simulink model "MR30Simulinknodos"  (R2013a)
settings: Solver=ode23tb  StartTime=0.0  StopTime=10.0  RelTol=1e-3
libraries: powerlib x200
(part 1 of 2)
settings Model: Creator=Erika  LastModifiedBy=Erika

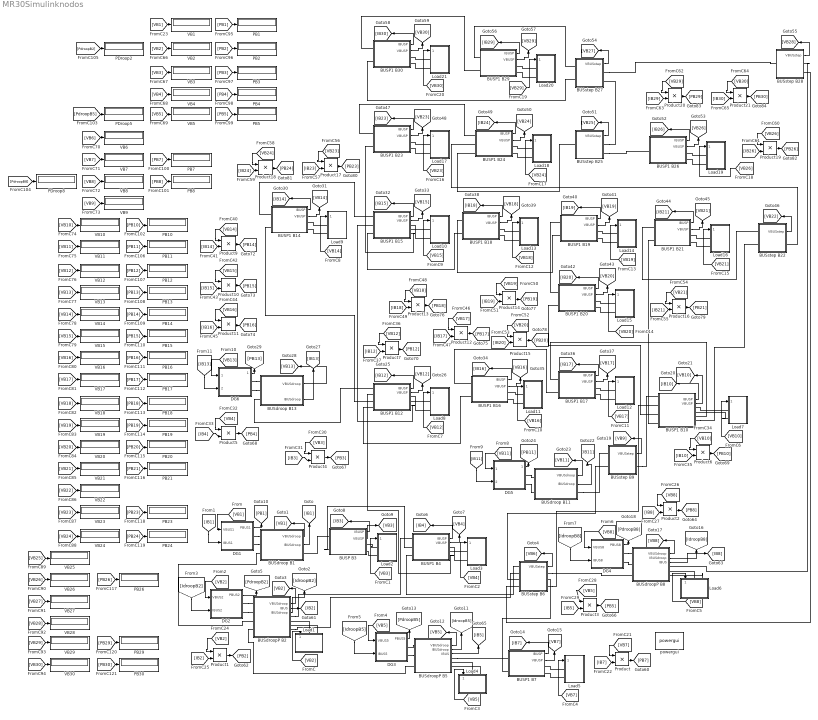
== system MR30Simulinknodos ==
  BUSP B3 : Subsystem
  BUSP1 B10 : Subsystem
  BUSP1 B12 : Subsystem
  BUSP1 B14 : Subsystem
  BUSP1 B15 : Subsystem
  BUSP1 B16 : Subsystem
  BUSP1 B17 : Subsystem
  BUSP1 B18 : Subsystem
  BUSP1 B19 : Subsystem
  BUSP1 B20 : Subsystem
  BUSP1 B21 : Subsystem
  BUSP1 B23 : Subsystem
  BUSP1 B24 : Subsystem
  BUSP1 B26 : Subsystem
  BUSP1 B29 : Subsystem
  BUSP1 B30 : Subsystem
  BUSP1 B4 : Subsystem
  BUSP1 B7 : Subsystem
  BUSdroop B1 : Subsystem
  BUSdroop B11 : Subsystem
  BUSdroop B13 : Subsystem
  BUSdroopP B2 : Subsystem
  BUSdroopP B5 : Subsystem
  BUSdroopP B8 : Subsystem
  BUSstep B22 : Subsystem
  BUSstep B25 : Subsystem
  BUSstep B27 : Subsystem
  BUSstep B28 : Subsystem
  BUSstep B6 : Subsystem
  BUSstep B9 : Subsystem
  DG1 : Subsystem
  DG2 : Subsystem
  DG3 : Subsystem
  DG4 : Subsystem
  DG5 : Subsystem
  DG6 : Subsystem
  Load1 : Subsystem
  Load10 : Subsystem
  Load11 : Subsystem
  Load12 : Subsystem
  Load13 : Subsystem
  Load14 : Subsystem
  Load15 : Subsystem
  Load16 : Subsystem
  Load17 : Subsystem
  Load18 : Subsystem
  Load19 : Subsystem
  Load2 : Subsystem
  Load20 : Subsystem
  Load21 : Subsystem
  Load3 : Subsystem
  Load4 : Subsystem
  Load5 : Subsystem
  Load6 : Subsystem
  Load7 : Subsystem
  Load8 : Subsystem
  Load9 : Subsystem
  PB{1..5,7..8,10..21,23..24,26,29..30} (24 alike) : Display
  PDroop2 : Display
  PDroop5 : Display
  PDroop8 : Display
  Product{,1..7,9..21} (21 alike) : Product
  VB{1..30} (30 alike) : Display
  powergui : powerlib/powergui  Priority=1  SimulationMode=Continuous  SolverType=Tustin  SampleTime=50e-6  frequency=60  SPID=off  DisableSnubberDevices=off  DisableRonSwitches=off  DisableVfSwitches=off  SwTol=0  Interpol=off  DisplayEquations=off  frequencyindice=0  Pbase=100e6  ErrMax=1e-4  Iterations=50  UnitsV=kV  UnitsW=MW  FunctionMessages=off  echomessages=off  HookPort=off  EnableUseOfTLC=off  x0status=blocks  RestoreLinks=warning  ResistiveCurrentMeasurement=off  Frange=[0:2:500]  Ylog=off  Xlog=on  ShowGrid=off  save=off  variable=ZData  ZoomFFT=off  StartTime=0.0  cycles=1  DisplayStyle=1  fundamental=60  FreqAxis=off  MaxFrequency=1000  frequencyindicesteady=1  RmsSteady=1  display=off  Ts=0  methode=off
  wires:
  BUSdroop B1/1(VBUSdroop) -> [VB1]
  BUSdroop B1/2(IBUSdroop) -> [IB1]
  [VB1] -> DG1/1(VBUS1)
  DG1/1(PBUS1) -> [PB1]
  BUSP B3/1(IBUSP) -> [IB3]
  BUSP B3/2(VBUSP) -> [VB3]
  [VB2] -> Load1/1(VBUSc)
  BUSdroopP B2/1(VBUSdroop) -> [VB2]
  BUSstep B6/1(VBUSstep) -> [VB6]
  [VB2] -> DG2/1(VBUS2)
  [IdroopB2] -> DG2/2(IBUS2)
  [VB3] -> Load2/1(VBUSc)
  BUSP1 B4/1(IBUSP) -> [IB4]
  BUSP1 B4/2(VBUSP) -> [VB4]
  [VB4] -> Load3/1(VBUSc)
  [VB5] -> Load4/1(VBUSc)
  BUSdroopP B5/1(VBUSdroop) -> [VB5]
  BUSdroopP B5/2(IBUSdroop) -> [IdroopB5]
  [VB5] -> DG3/1(VBUS5)
  [IdroopB5] -> DG3/2(IBUS5)
  DG3/1(PBUS5) -> [PdroopB5]
  BUSP1 B7/1(IBUSP) -> [IB7]
  BUSP1 B7/2(VBUSP) -> [VB7]
  [VB7] -> Load5/1(VBUSc)
  [VB8] -> Load6/1(VBUSc)
  BUSdroopP B8/1(VBUSdroop) -> [VB8]
  BUSdroopP B8/2(IBUSdroop) -> [IdroopB8]
  [VB8] -> DG4/1(VBUS8)
  [IdroopB8] -> DG4/2(IBUS8)
  DG4/1(PBUS8) -> [PdroopB8]
  BUSstep B9/1(VBUSstep) -> [VB9]
  BUSP1 B10/1(IBUSP) -> [IB10]
  BUSP1 B10/2(VBUSP) -> [VB10]
  [VB10] -> Load7/1(VBUSc)
  BUSdroop B11/1(VBUSdroop) -> [VB11]
  BUSdroop B11/2(IBUSdroop) -> [IB11]
  [VB11] -> DG5/1(VBUS11)
  [IB11] -> DG5/2(IBUS11)
  DG5/1(PBUS11) -> [PB11]
  BUSP1 B12/1(IBUSP) -> [IB12]
  BUSP1 B12/2(VBUSP) -> [VB12]
  [VB12] -> Load8/1(VBUSc)
  BUSdroop B13/1(VBUSdroop) -> [VB13]
  BUSdroop B13/2(IBUSdroop) -> [IB13]
  [VB13] -> DG6/1(VBUS13)
  [IB13] -> DG6/2(IBUS13)
  DG6/1(PBUS13) -> [PB13]
  BUSP1 B14/1(IBUSP) -> [IB14]
  BUSP1 B14/2(VBUSP) -> [VB14]
  [VB14] -> Load9/1(VBUSc)
  BUSP1 B15/1(IBUSP) -> [IB15]
  BUSP1 B15/2(VBUSP) -> [VB15]
  [VB15] -> Load10/1(VBUSc)
  BUSP1 B16/1(IBUSP) -> [IB16]
  BUSP1 B16/2(VBUSP) -> [VB16]
  [VB16] -> Load11/1(VBUSc)
  BUSP1 B17/1(IBUSP) -> [IB17]
  BUSP1 B17/2(VBUSP) -> [VB17]
  [VB17] -> Load12/1(VBUSc)
  BUSP1 B18/1(IBUSP) -> [IB18]
  BUSP1 B18/2(VBUSP) -> [VB18]
  [VB18] -> Load13/1(VBUSc)
  BUSP1 B19/1(IBUSP) -> [IB19]
  BUSP1 B19/2(VBUSP) -> [VB19]
  [VB19] -> Load14/1(VBUSc)
  BUSP1 B20/1(IBUSP) -> [IB20]
  BUSP1 B20/2(VBUSP) -> [VB20]
  [VB20] -> Load15/1(VBUSc)
  BUSP1 B21/1(IBUSP) -> [IB21]
  BUSP1 B21/2(VBUSP) -> [VB21]
  [VB21] -> Load16/1(VBUSc)
  BUSstep B22/1(VBUSstep) -> [VB22]
  BUSP1 B23/1(IBUSP) -> [IB23]
  BUSP1 B23/2(VBUSP) -> [VB23]
  [VB23] -> Load17/1(VBUSc)
  BUSP1 B24/1(IBUSP) -> [IB24]
  BUSP1 B24/2(VBUSP) -> [VB24]
  [VB24] -> Load18/1(VBUSc)
  BUSstep B25/1(VBUSstep) -> [VB25]
  BUSP1 B26/1(IBUSP) -> [IB26]
  BUSP1 B26/2(VBUSP) -> [VB26]
  [VB26] -> Load19/1(VBUSc)
  BUSstep B27/1(VBUSstep) -> [VB27]
  BUSstep B28/1(VBUSstep) -> [VB28]
  BUSP1 B29/1(IBUSP) -> [IB29]
  BUSP1 B29/2(VBUSP) -> [VB29]
  [VB29] -> Load20/1(VBUSc)
  BUSP1 B30/1(IBUSP) -> [IB30]
  BUSP1 B30/2(VBUSP) -> [VB30]
  [VB30] -> Load21/1(VBUSc)
  [IB1] -> DG1/2(IBUS1)
  Product/1 -> [PB7]
  [IB7] -> Product/2
  [VB7] -> Product/1
  DG2/1(PBUS2) -> [PdroopB2]
  Product1/1 -> [PB2]
  [IB2] -> Product1/2
  [VB2] -> Product1/1
  BUSdroopP B2/3(IBUSdroop) -> [IdroopB2]
  BUSdroopP B2/2(IBUS) -> [IB2]
  BUSdroopP B8/3(IBUS) -> [IB8]
  Product2/1 -> [PB8]
  [IB8] -> Product2/2
  [VB8] -> Product2/1
  BUSdroopP B5/3(IBUS) -> [IB5]
  Product3/1 -> [PB5]
  [IB5] -> Product3/2
  [VB5] -> Product3/1
  Product4/1 -> [PB3]
  [IB3] -> Product4/2
  [VB3] -> Product4/1
  Product5/1 -> [PB4]
  [IB4] -> Product5/2
  [VB4] -> Product5/1
  Product6/1 -> [PB10]
  [IB10] -> Product6/2
  [VB10] -> Product6/1
  Product7/1 -> [PB12]
  [IB12] -> Product7/2
  [VB12] -> Product7/1
  Product9/1 -> [PB14]
  [IB14] -> Product9/2
  [VB14] -> Product9/1
  Product10/1 -> [PB15]
  [IB15] -> Product10/2
  [VB15] -> Product10/1
  Product11/1 -> [PB16]
  [IB16] -> Product11/2
  [VB16] -> Product11/1
  Product12/1 -> [PB17]
  [IB17] -> Product12/2
  [VB17] -> Product12/1
  Product13/1 -> [PB18]
  [IB18] -> Product13/2
  [VB18] -> Product13/1
  Product14/1 -> [PB19]
  [IB19] -> Product14/2
  [VB19] -> Product14/1
  Product15/1 -> [PB20]
  [IB20] -> Product15/2
  [VB20] -> Product15/1
  Product16/1 -> [PB21]
  [IB21] -> Product16/2
  [VB21] -> Product16/1
  Product17/1 -> [PB23]
  [IB23] -> Product17/2
  [VB23] -> Product17/1
  Product18/1 -> [PB24]
  [IB24] -> Product18/2
  [VB24] -> Product18/1
  Product19/1 -> [PB26]
  [IB26] -> Product19/2
  [VB26] -> Product19/1
  Product20/1 -> [PB29]
  [IB29] -> Product20/2
  [VB29] -> Product20/1
  Product21/1 -> [PB30]
  [IB30] -> Product21/2
  [VB30] -> Product21/1
  [VB1] -> VB1/1
  [VB2] -> VB2/1
  [VB3] -> VB3/1
  [VB5] -> VB5/1
  [VB6] -> VB6/1
  [VB7] -> VB7/1
  [VB8] -> VB8/1
  [VB9] -> VB9/1
  [VB10] -> VB10/1
  [VB11] -> VB11/1
  [VB12] -> VB12/1
  [VB13] -> VB13/1
  [VB14] -> VB14/1
  [VB15] -> VB15/1
  [VB16] -> VB16/1
  [VB17] -> VB17/1
  [VB18] -> VB18/1
  [VB19] -> VB19/1
  [VB20] -> VB20/1
  [VB21] -> VB21/1
  [VB22] -> VB22/1
  [VB23] -> VB23/1
  [VB24] -> VB24/1
  [VB25] -> VB25/1
  [VB26] -> VB26/1
  [VB27] -> VB27/1
  [VB28] -> VB28/1
  [VB29] -> VB29/1
  [VB30] -> VB30/1
  [PB1] -> PB1/1
  [PB2] -> PB2/1
  [PB3] -> PB3/1
  [PB4] -> PB4/1
  [PB5] -> PB5/1
  [PB8] -> PB8/1
  [PB10] -> PB10/1
  [PdroopB5] -> PDroop5/1
  [PdroopB8] -> PDroop8/1
  [PdroopB2] -> PDroop2/1
  [PB12] -> PB12/1
  [PB13] -> PB13/1
  [PB14] -> PB14/1
  [PB15] -> PB15/1
  [PB16] -> PB16/1
  [PB17] -> PB17/1
  [PB18] -> PB18/1
  [PB19] -> PB19/1
  [PB20] -> PB20/1
  [PB21] -> PB21/1
  [PB23] -> PB23/1
  [PB24] -> PB24/1
  [PB26] -> PB26/1
  [PB29] -> PB29/1
  [PB30] -> PB30/1
  [PB11] -> PB11/1
  [PB7] -> PB7/1
  [VB4] -> VB4/1
  connections:
  DG1/RConn1 -- BUSdroop B1/LConn1
  DG1/RConn2 -- BUSdroop B1/LConn2
  DG2/RConn1 -- BUSdroopP B2/LConn1
  DG2/RConn2 -- BUSdroopP B2/LConn2
  Load1/LConn1 -- BUSdroopP B2/RConn2
  Load1/LConn2 -- BUSdroopP B2/RConn3
  Load2/LConn1 -- BUSP B3/RConn1
  Load2/LConn2 -- BUSP B3/RConn2
  Load3/LConn2 -- BUSP1 B4/RConn2
  Load3/LConn1 -- BUSP1 B4/RConn1
  DG3/RConn1 -- BUSdroopP B5/LConn1
  DG3/RConn2 -- BUSdroopP B5/LConn2
  Load4/LConn1 -- BUSdroopP B5/RConn2
  Load4/LConn2 -- BUSdroopP B5/RConn3
  Load5/LConn1 -- BUSP1 B7/RConn1
  Load5/LConn2 -- BUSP1 B7/RConn2
  Load6/LConn2 -- BUSdroopP B8/RConn3
  DG4/RConn1 -- BUSdroopP B8/LConn1
  DG4/RConn2 -- BUSdroopP B8/LConn2
  Load6/LConn1 -- BUSdroopP B8/RConn2
  Load7/LConn2 -- BUSP1 B10/RConn2
  Load7/LConn1 -- BUSP1 B10/RConn1
  DG5/RConn1 -- BUSdroop B11/LConn1
  DG5/RConn2 -- BUSdroop B11/LConn2
  Load8/LConn2 -- BUSP1 B12/RConn2
  Load8/LConn1 -- BUSP1 B12/RConn1
  DG6/RConn2 -- BUSdroop B13/LConn2
  DG6/RConn1 -- BUSdroop B13/LConn1
  Load9/LConn2 -- BUSP1 B14/RConn2
  Load9/LConn1 -- BUSP1 B14/RConn1
  Load10/LConn1 -- BUSP1 B15/RConn1
  Load10/LConn2 -- BUSP1 B15/RConn2
  Load11/LConn2 -- BUSP1 B16/RConn2
  Load11/LConn1 -- BUSP1 B16/RConn1
  Load12/LConn2 -- BUSP1 B17/RConn2
  Load12/LConn1 -- BUSP1 B17/RConn1
  Load13/LConn2 -- BUSP1 B18/RConn2
  Load13/LConn1 -- BUSP1 B18/RConn1
  Load14/LConn1 -- BUSP1 B19/RConn1
  Load14/LConn2 -- BUSP1 B19/RConn2
  Load15/LConn1 -- BUSP1 B20/RConn1
  Load15/LConn2 -- BUSP1 B20/RConn2
  Load16/LConn1 -- BUSP1 B21/RConn1
  Load16/LConn2 -- BUSP1 B21/RConn2
  Load17/LConn2 -- BUSP1 B23/RConn2
  Load17/LConn1 -- BUSP1 B23/RConn1
  Load18/LConn2 -- BUSP1 B24/RConn2
  Load18/LConn1 -- BUSP1 B24/RConn1
  Load19/LConn2 -- BUSP1 B26/RConn2
  Load19/LConn1 -- BUSP1 B26/RConn1
  Load20/LConn1 -- BUSP1 B29/RConn1
  Load20/LConn2 -- BUSP1 B29/RConn2
  Load21/LConn2 -- BUSP1 B30/RConn2
  Load21/LConn1 -- BUSP1 B30/RConn1
  BUSdroopP B2/LConn3 -- BUSdroop B1/LConn3
  BUSP B3/LConn1 -- BUSdroop B1/RConn1
  BUSdroopP B2/RConn1 -- BUSP1 B4/LConn1
  BUSP B3/LConn2 -- BUSP1 B4/LConn2
  BUSdroopP B2/LConn4 -- BUSdroopP B5/LConn3
  BUSdroopP B2/RConn4 -- BUSstep B6/LConn2
  BUSP1 B4/LConn3 -- BUSstep B6/LConn1
  BUSdroopP B5/RConn1 -- BUSP1 B7/LConn1
  BUSP1 B7/LConn2 -- BUSstep B6/RConn2
  BUSstep B6/RConn1 -- BUSdroopP B8/LConn3
  BUSstep B6/LConn3 -- BUSstep B9/LConn2
  BUSstep B6/RConn3 -- BUSP1 B10/LConn2
  BUSdroop B11/RConn1 -- BUSstep B9/LConn1
  BUSstep B9/RConn1 -- BUSP1 B10/LConn1
  BUSP1 B4/RConn3 -- BUSP1 B12/LConn2
  BUSdroop B13/LConn3 -- BUSP1 B12/LConn1
  BUSP1 B14/LConn2 -- BUSP1 B12/LConn3
  BUSP1 B12/RConn3 -- BUSP1 B15/LConn2
  BUSP1 B12/LConn4 -- BUSP1 B16/LConn2
  BUSP1 B14/LConn1 -- BUSP1 B15/LConn1
  BUSP1 B16/LConn1 -- BUSP1 B17/LConn2
  BUSP1 B15/LConn3 -- BUSP1 B18/LConn2
  BUSP1 B18/LConn1 -- BUSP1 B19/LConn2
  BUSP1 B20/LConn1 -- BUSP1 B19/LConn1
  BUSP1 B20/LConn2 -- BUSP1 B10/LConn3
  BUSP1 B17/LConn1 -- BUSP1 B10/RConn3
  BUSP1 B21/LConn2 -- BUSP1 B10/LConn4
  BUSP1 B10/RConn4 -- BUSstep B22/LConn2
  BUSP1 B21/LConn1 -- BUSstep B22/LConn1
  BUSP1 B15/RConn3 -- BUSP1 B23/LConn2
  BUSP1 B24/LConn2 -- BUSstep B22/RConn1
  BUSP1 B23/LConn1 -- BUSP1 B24/LConn1
  BUSP1 B24/LConn3 -- BUSstep B25/LConn1
  BUSstep B25/RConn2 -- BUSP1 B26/LConn1
  BUSstep B25/RConn1 -- BUSstep B27/RConn2
  BUSstep B27/RConn1 -- BUSstep B28/LConn1
  BUSstep B27/LConn1 -- BUSP1 B29/LConn1
  BUSP1 B30/LConn2 -- BUSstep B27/LConn2
  BUSP1 B30/LConn1 -- BUSP1 B29/LConn2
  BUSstep B28/RConn1 -- BUSdroopP B8/RConn1
  BUSstep B6/LConn4 -- BUSstep B28/RConn2

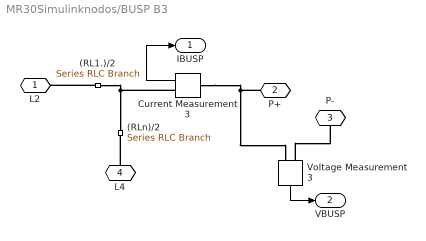
== system MR30Simulinknodos/BUSP B3 ==
  (RL1.)/2 : powerlib/Elements/Series RLC Branch  LConnTagsString=__new0  RConnTagsString=__new0  BranchType=R  Resistance=0.645456/2  Inductance=1e-3  SetiL0=off  InitialCurrent=0  Capacitance=1e-6  Setx0=off  InitialVoltage=0  Measurements=None
  (RLn)/2 : powerlib/Elements/Series RLC Branch  LConnTagsString=__new0  RConnTagsString=__new0  BranchType=R  Resistance=.188496/2  Inductance=1e-3  SetiL0=off  InitialCurrent=0  Capacitance=1e-6  Setx0=off  InitialVoltage=0  Measurements=None
  Current Measurement3 : powerlib/Measurements/Current Measurement  PhasorSimulation=off  OutputType=Complex  PSBequivalent=0
  Voltage Measurement3 : powerlib/Measurements/Voltage Measurement  PhasorSimulation=off  OutputType=Complex  PSBequivalent=0
  L2 : PMIOPort  Port=1  Side=Left
  P+ : PMIOPort  Port=2  Side=Right
  P- : PMIOPort  Port=3  Side=Right
  L4 : PMIOPort  Port=4  Side=Left
  IBUSP : Outport
  VBUSP : Outport  Port=2
  wires:
  Voltage Measurement3/1 -> VBUSP/1
  Current Measurement3/1 -> IBUSP/1
  connections:
  P+/RConn1 -- Voltage Measurement3/LConn1 -- Current Measurement3/LConn1
  (RL1.)/2/RConn1 -- Current Measurement3/RConn1 -- (RLn)/2/LConn1
  (RL1.)/2/LConn1 -- L2/RConn1
  L4/RConn1 -- (RLn)/2/RConn1
  Voltage Measurement3/LConn2 -- P-/RConn1

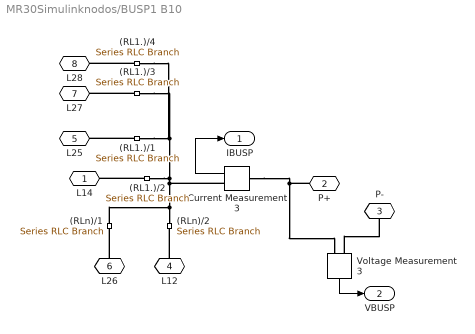
== system MR30Simulinknodos/BUSP1 B10 ==
  (RL1.)/1 : powerlib/Elements/Series RLC Branch  LConnTagsString=__new0  RConnTagsString=__new0  BranchType=R  Resistance=1.336608/2  Inductance=1e-3  SetiL0=off  InitialCurrent=0  Capacitance=1e-6  Setx0=off  InitialVoltage=0  Measurements=None
  (RL1.)/2 : powerlib/Elements/Series RLC Branch  LConnTagsString=__new0  RConnTagsString=__new0  BranchType=R  Resistance=1.5708/2  Inductance=1e-3  SetiL0=off  InitialCurrent=0  Capacitance=1e-6  Setx0=off  InitialVoltage=0  Measurements=None
  (RL1.)/3 : powerlib/Elements/Series RLC Branch  LConnTagsString=__new0  RConnTagsString=__new0  BranchType=R  Resistance=0.496944/2  Inductance=1e-3  SetiL0=off  InitialCurrent=0  Capacitance=1e-6  Setx0=off  InitialVoltage=0  Measurements=None
  (RL1.)/4 : powerlib/Elements/Series RLC Branch  LConnTagsString=__new0  RConnTagsString=__new0  BranchType=R  Resistance=1.038156/2  Inductance=1e-3  SetiL0=off  InitialCurrent=0  Capacitance=1e-6  Setx0=off  InitialVoltage=0  Measurements=None
  (RLn)/1 : powerlib/Elements/Series RLC Branch  LConnTagsString=__new0  RConnTagsString=__new0  BranchType=R  Resistance=0.462672/2  Inductance=1e-3  SetiL0=off  InitialCurrent=0  Capacitance=1e-6  Setx0=off  InitialVoltage=0  Measurements=None
  (RLn)/2 : powerlib/Elements/Series RLC Branch  LConnTagsString=__new0  RConnTagsString=__new0  BranchType=R  Resistance=7.93968/2  Inductance=1e-3  SetiL0=off  InitialCurrent=0  Capacitance=1e-6  Setx0=off  InitialVoltage=0  Measurements=None
  Current Measurement3 : powerlib/Measurements/Current Measurement  PhasorSimulation=off  OutputType=Complex  PSBequivalent=0
  Voltage Measurement3 : powerlib/Measurements/Voltage Measurement  PhasorSimulation=off  OutputType=Complex  PSBequivalent=0
  L14 : PMIOPort  Port=1  Side=Left
  P+ : PMIOPort  Port=2  Side=Right
  P- : PMIOPort  Port=3  Side=Right
  L12 : PMIOPort  Port=4  Side=Left
  L25 : PMIOPort  Port=5  Side=Left
  L26 : PMIOPort  Port=6  Side=Right
  L27 : PMIOPort  Port=7  Side=Left
  L28 : PMIOPort  Port=8  Side=Right
  IBUSP : Outport
  VBUSP : Outport  Port=2
  wires:
  Current Measurement3/1 -> IBUSP/1
  Voltage Measurement3/1 -> VBUSP/1
  connections:
  Voltage Measurement3/LConn2 -- P-/RConn1
  L12/RConn1 -- (RLn)/2/RConn1
  (RL1.)/2/LConn1 -- L14/RConn1
  (RL1.)/4/RConn1 -- (RL1.)/3/RConn1 -- (RL1.)/1/RConn1 -- (RL1.)/2/RConn1 -- Current Measurement3/RConn1 -- (RLn)/1/LConn1 -- (RLn)/2/LConn1
  Current Measurement3/LConn1 -- Voltage Measurement3/LConn1 -- P+/RConn1
  (RL1.)/1/LConn1 -- L25/RConn1
  L26/RConn1 -- (RLn)/1/RConn1
  (RL1.)/3/LConn1 -- L27/RConn1
  (RL1.)/4/LConn1 -- L28/RConn1

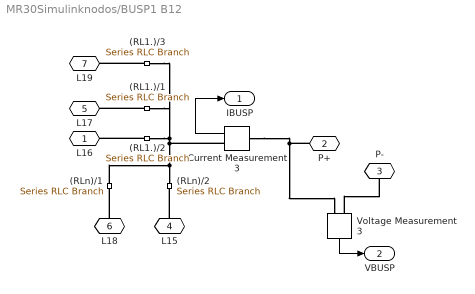
== system MR30Simulinknodos/BUSP1 B12 ==
  (RL1.)/1 : powerlib/Elements/Series RLC Branch  LConnTagsString=__new0  RConnTagsString=__new0  BranchType=R  Resistance=1.757868/2  Inductance=1e-3  SetiL0=off  InitialCurrent=0  Capacitance=1e-6  Setx0=off  InitialVoltage=0  Measurements=None
  (RL1.)/2 : powerlib/Elements/Series RLC Branch  LConnTagsString=__new0  RConnTagsString=__new0  BranchType=R  Resistance=1.9992/2  Inductance=1e-3  SetiL0=off  InitialCurrent=0  Capacitance=1e-6  Setx0=off  InitialVoltage=0  Measurements=None
  (RL1.)/3 : powerlib/Elements/Series RLC Branch  LConnTagsString=__new0  RConnTagsString=__new0  BranchType=R  Resistance=1.34946/2  Inductance=1e-3  SetiL0=off  InitialCurrent=0  Capacitance=1e-6  Setx0=off  InitialVoltage=0  Measurements=None
  (RLn)/1 : powerlib/Elements/Series RLC Branch  LConnTagsString=__new0  RConnTagsString=__new0  BranchType=R  Resistance=0.945336/2  Inductance=1e-3  SetiL0=off  InitialCurrent=0  Capacitance=1e-6  Setx0=off  InitialVoltage=0  Measurements=None
  (RLn)/2 : powerlib/Elements/Series RLC Branch  LConnTagsString=__new0  RConnTagsString=__new0  BranchType=R  Resistance=3.65568/2  Inductance=1e-3  SetiL0=off  InitialCurrent=0  Capacitance=1e-6  Setx0=off  InitialVoltage=0  Measurements=None
  Current Measurement3 : powerlib/Measurements/Current Measurement  PhasorSimulation=off  OutputType=Complex  PSBequivalent=0
  Voltage Measurement3 : powerlib/Measurements/Voltage Measurement  PhasorSimulation=off  OutputType=Complex  PSBequivalent=0
  L16 : PMIOPort  Port=1  Side=Left
  P+ : PMIOPort  Port=2  Side=Right
  P- : PMIOPort  Port=3  Side=Right
  L15 : PMIOPort  Port=4  Side=Left
  L17 : PMIOPort  Port=5  Side=Left
  L18 : PMIOPort  Port=6  Side=Right
  L19 : PMIOPort  Port=7  Side=Left
  IBUSP : Outport
  VBUSP : Outport  Port=2
  wires:
  Voltage Measurement3/1 -> VBUSP/1
  Current Measurement3/1 -> IBUSP/1
  connections:
  P+/RConn1 -- Voltage Measurement3/LConn1 -- Current Measurement3/LConn1
  (RL1.)/2/RConn1 -- (RL1.)/3/RConn1 -- (RL1.)/1/RConn1 -- Current Measurement3/RConn1 -- (RLn)/1/LConn1 -- (RLn)/2/LConn1
  (RL1.)/2/LConn1 -- L16/RConn1
  L15/RConn1 -- (RLn)/2/RConn1
  Voltage Measurement3/LConn2 -- P-/RConn1
  (RL1.)/1/LConn1 -- L17/RConn1
  L18/RConn1 -- (RLn)/1/RConn1
  (RL1.)/3/LConn1 -- L19/RConn1

== system MR30Simulinknodos/BUSP1 B14 ==
  (RL1.)/2 : powerlib/Elements/Series RLC Branch  LConnTagsString=__new0  RConnTagsString=__new0  BranchType=R  Resistance=3.15588/2  Inductance=1e-3  SetiL0=off  InitialCurrent=0  Capacitance=1e-6  Setx0=off  InitialVoltage=0  Measurements=None
  (RLn)/2 : powerlib/Elements/Series RLC Branch  LConnTagsString=__new0  RConnTagsString=__new0  BranchType=R  Resistance=1.757868/2  Inductance=1e-3  SetiL0=off  InitialCurrent=0  Capacitance=1e-6  Setx0=off  InitialVoltage=0  Measurements=None
  Current Measurement3 : powerlib/Measurements/Current Measurement  PhasorSimulation=off  OutputType=Complex  PSBequivalent=0
  Voltage Measurement3 : powerlib/Measurements/Voltage Measurement  PhasorSimulation=off  OutputType=Complex  PSBequivalent=0
  L20 : PMIOPort  Port=1  Side=Left
  P+ : PMIOPort  Port=2  Side=Right
  P- : PMIOPort  Port=3  Side=Right
  L17 : PMIOPort  Port=4  Side=Left
  IBUSP : Outport
  VBUSP : Outport  Port=2
  wires:
  Current Measurement3/1 -> IBUSP/1
  Voltage Measurement3/1 -> VBUSP/1
  connections:
  Voltage Measurement3/LConn2 -- P-/RConn1
  L17/RConn1 -- (RLn)/2/RConn1
  (RL1.)/2/LConn1 -- L20/RConn1
  (RLn)/2/LConn1 -- Current Measurement3/RConn1 -- (RL1.)/2/RConn1
  Current Measurement3/LConn1 -- Voltage Measurement3/LConn1 -- P+/RConn1

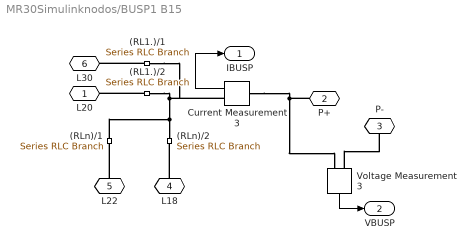
== system MR30Simulinknodos/BUSP1 B15 ==
  (RL1.)/1 : powerlib/Elements/Series RLC Branch  LConnTagsString=__new0  RConnTagsString=__new0  BranchType=R  Resistance=1.428/2  Inductance=1e-3  SetiL0=off  InitialCurrent=0  Capacitance=1e-6  Setx0=off  InitialVoltage=0  Measurements=None
  (RL1.)/2 : powerlib/Elements/Series RLC Branch  LConnTagsString=__new0  RConnTagsString=__new0  BranchType=R  Resistance=3.15588/2  Inductance=1e-3  SetiL0=off  InitialCurrent=0  Capacitance=1e-6  Setx0=off  InitialVoltage=0  Measurements=None
  (RLn)/1 : powerlib/Elements/Series RLC Branch  LConnTagsString=__new0  RConnTagsString=__new0  BranchType=R  Resistance=1.52796/2  Inductance=1e-3  SetiL0=off  InitialCurrent=0  Capacitance=1e-6  Setx0=off  InitialVoltage=0  Measurements=None
  (RLn)/2 : powerlib/Elements/Series RLC Branch  LConnTagsString=__new0  RConnTagsString=__new0  BranchType=R  Resistance=0.945336/2  Inductance=1e-3  SetiL0=off  InitialCurrent=0  Capacitance=1e-6  Setx0=off  InitialVoltage=0  Measurements=None
  Current Measurement3 : powerlib/Measurements/Current Measurement  PhasorSimulation=off  OutputType=Complex  PSBequivalent=0
  Voltage Measurement3 : powerlib/Measurements/Voltage Measurement  PhasorSimulation=off  OutputType=Complex  PSBequivalent=0
  L20 : PMIOPort  Port=1  Side=Left
  P+ : PMIOPort  Port=2  Side=Right
  P- : PMIOPort  Port=3  Side=Right
  L18 : PMIOPort  Port=4  Side=Left
  L22 : PMIOPort  Port=5  Side=Left
  L30 : PMIOPort  Port=6  Side=Right
  IBUSP : Outport
  VBUSP : Outport  Port=2
  wires:
  Voltage Measurement3/1 -> VBUSP/1
  Current Measurement3/1 -> IBUSP/1
  connections:
  P+/RConn1 -- Voltage Measurement3/LConn1 -- Current Measurement3/LConn1
  (RL1.)/2/RConn1 -- (RL1.)/1/RConn1 -- Current Measurement3/RConn1 -- (RLn)/1/LConn1 -- (RLn)/2/LConn1
  (RL1.)/2/LConn1 -- L20/RConn1
  L18/RConn1 -- (RLn)/2/RConn1
  Voltage Measurement3/LConn2 -- P-/RConn1
  L22/RConn1 -- (RLn)/1/RConn1
  (RL1.)/1/LConn1 -- L30/RConn1

== system MR30Simulinknodos/BUSP1 B16 ==
  (RL1.)/2 : powerlib/Elements/Series RLC Branch  LConnTagsString=__new0  RConnTagsString=__new0  BranchType=R  Resistance=1.176672/2  Inductance=1e-3  SetiL0=off  InitialCurrent=0  Capacitance=1e-6  Setx0=off  InitialVoltage=0  Measurements=None
  (RLn)/2 : powerlib/Elements/Series RLC Branch  LConnTagsString=__new0  RConnTagsString=__new0  BranchType=R  Resistance=1.34946/2  Inductance=1e-3  SetiL0=off  InitialCurrent=0  Capacitance=1e-6  Setx0=off  InitialVoltage=0  Measurements=None
  Current Measurement3 : powerlib/Measurements/Current Measurement  PhasorSimulation=off  OutputType=Complex  PSBequivalent=0
  Voltage Measurement3 : powerlib/Measurements/Voltage Measurement  PhasorSimulation=off  OutputType=Complex  PSBequivalent=0
  L21 : PMIOPort  Port=1  Side=Left
  P+ : PMIOPort  Port=2  Side=Right
  P- : PMIOPort  Port=3  Side=Right
  L19 : PMIOPort  Port=4  Side=Left
  IBUSP : Outport
  VBUSP : Outport  Port=2
  wires:
  Current Measurement3/1 -> IBUSP/1
  Voltage Measurement3/1 -> VBUSP/1
  connections:
  Voltage Measurement3/LConn2 -- P-/RConn1
  L19/RConn1 -- (RLn)/2/RConn1
  (RL1.)/2/LConn1 -- L21/RConn1
  (RLn)/2/LConn1 -- Current Measurement3/RConn1 -- (RL1.)/2/RConn1
  Current Measurement3/LConn1 -- Voltage Measurement3/LConn1 -- P+/RConn1

== system MR30Simulinknodos/BUSP1 B17 ==
  (RL1.)/2 : powerlib/Elements/Series RLC Branch  LConnTagsString=__new0  RConnTagsString=__new0  BranchType=R  Resistance=0.462672/2  Inductance=1e-3  SetiL0=off  InitialCurrent=0  Capacitance=1e-6  Setx0=off  InitialVoltage=0  Measurements=None
  (RLn)/2 : powerlib/Elements/Series RLC Branch  LConnTagsString=__new0  RConnTagsString=__new0  BranchType=R  Resistance=1.176672/2  Inductance=1e-3  SetiL0=off  InitialCurrent=0  Capacitance=1e-6  Setx0=off  InitialVoltage=0  Measurements=None
  Current Measurement3 : powerlib/Measurements/Current Measurement  PhasorSimulation=off  OutputType=Complex  PSBequivalent=0
  Voltage Measurement3 : powerlib/Measurements/Voltage Measurement  PhasorSimulation=off  OutputType=Complex  PSBequivalent=0
  L26 : PMIOPort  Port=1  Side=Left
  P+ : PMIOPort  Port=2  Side=Right
  P- : PMIOPort  Port=3  Side=Right
  L21 : PMIOPort  Port=4  Side=Left
  IBUSP : Outport
  VBUSP : Outport  Port=2
  wires:
  Voltage Measurement3/1 -> VBUSP/1
  Current Measurement3/1 -> IBUSP/1
  connections:
  P+/RConn1 -- Voltage Measurement3/LConn1 -- Current Measurement3/LConn1
  (RL1.)/2/RConn1 -- Current Measurement3/RConn1 -- (RLn)/2/LConn1
  (RL1.)/2/LConn1 -- L26/RConn1
  L21/RConn1 -- (RLn)/2/RConn1
  Voltage Measurement3/LConn2 -- P-/RConn1

== system MR30Simulinknodos/BUSP1 B18 ==
  (RL1.)/2 : powerlib/Elements/Series RLC Branch  LConnTagsString=__new0  RConnTagsString=__new0  BranchType=R  Resistance=0.912492/2  Inductance=1e-3  SetiL0=off  InitialCurrent=0  Capacitance=1e-6  Setx0=off  InitialVoltage=0  Measurements=None
  (RLn)/2 : powerlib/Elements/Series RLC Branch  LConnTagsString=__new0  RConnTagsString=__new0  BranchType=R  Resistance=1.52796/2  Inductance=1e-3  SetiL0=off  InitialCurrent=0  Capacitance=1e-6  Setx0=off  InitialVoltage=0  Measurements=None
  Current Measurement3 : powerlib/Measurements/Current Measurement  PhasorSimulation=off  OutputType=Complex  PSBequivalent=0
  Voltage Measurement3 : powerlib/Measurements/Voltage Measurement  PhasorSimulation=off  OutputType=Complex  PSBequivalent=0
  L23 : PMIOPort  Port=1  Side=Left
  P+ : PMIOPort  Port=2  Side=Right
  P- : PMIOPort  Port=3  Side=Right
  L22 : PMIOPort  Port=4  Side=Left
  IBUSP : Outport
  VBUSP : Outport  Port=2
  wires:
  Current Measurement3/1 -> IBUSP/1
  Voltage Measurement3/1 -> VBUSP/1
  connections:
  Voltage Measurement3/LConn2 -- P-/RConn1
  L22/RConn1 -- (RLn)/2/RConn1
  (RL1.)/2/LConn1 -- L23/RConn1
  (RLn)/2/LConn1 -- Current Measurement3/RConn1 -- (RL1.)/2/RConn1
  Current Measurement3/LConn1 -- Voltage Measurement3/LConn1 -- P+/RConn1

== system MR30Simulinknodos/BUSP1 B19 ==
  (RL1.)/2 : powerlib/Elements/Series RLC Branch  LConnTagsString=__new0  RConnTagsString=__new0  BranchType=R  Resistance=4.8552/2  Inductance=1e-3  SetiL0=off  InitialCurrent=0  Capacitance=1e-6  Setx0=off  InitialVoltage=0  Measurements=None
  (RLn)/2 : powerlib/Elements/Series RLC Branch  LConnTagsString=__new0  RConnTagsString=__new0  BranchType=R  Resistance=0.912492/2  Inductance=1e-3  SetiL0=off  InitialCurrent=0  Capacitance=1e-6  Setx0=off  InitialVoltage=0  Measurements=None
  Current Measurement3 : powerlib/Measurements/Current Measurement  PhasorSimulation=off  OutputType=Complex  PSBequivalent=0
  Voltage Measurement3 : powerlib/Measurements/Voltage Measurement  PhasorSimulation=off  OutputType=Complex  PSBequivalent=0
  L24 : PMIOPort  Port=1  Side=Left
  P+ : PMIOPort  Port=2  Side=Right
  P- : PMIOPort  Port=3  Side=Right
  L23 : PMIOPort  Port=4  Side=Left
  IBUSP : Outport
  VBUSP : Outport  Port=2
  wires:
  Voltage Measurement3/1 -> VBUSP/1
  Current Measurement3/1 -> IBUSP/1
  connections:
  P+/RConn1 -- Voltage Measurement3/LConn1 -- Current Measurement3/LConn1
  (RL1.)/2/RConn1 -- Current Measurement3/RConn1 -- (RLn)/2/LConn1
  (RL1.)/2/LConn1 -- L24/RConn1
  L23/RConn1 -- (RLn)/2/RConn1
  Voltage Measurement3/LConn2 -- P-/RConn1

== system MR30Simulinknodos/BUSP1 B20 ==
  (RL1.)/2 : powerlib/Elements/Series RLC Branch  LConnTagsString=__new0  RConnTagsString=__new0  BranchType=R  Resistance=4.8552/2  Inductance=1e-3  SetiL0=off  InitialCurrent=0  Capacitance=1e-6  Setx0=off  InitialVoltage=0  Measurements=None
  (RLn)/2 : powerlib/Elements/Series RLC Branch  LConnTagsString=__new0  RConnTagsString=__new0  BranchType=R  Resistance=1.336608/2  Inductance=1e-3  SetiL0=off  InitialCurrent=0  Capacitance=1e-6  Setx0=off  InitialVoltage=0  Measurements=None
  Current Measurement3 : powerlib/Measurements/Current Measurement  PhasorSimulation=off  OutputType=Complex  PSBequivalent=0
  Voltage Measurement3 : powerlib/Measurements/Voltage Measurement  PhasorSimulation=off  OutputType=Complex  PSBequivalent=0
  L24 : PMIOPort  Port=1  Side=Left
  P+ : PMIOPort  Port=2  Side=Right
  P- : PMIOPort  Port=3  Side=Right
  L25 : PMIOPort  Port=4  Side=Left
  IBUSP : Outport
  VBUSP : Outport  Port=2
  wires:
  Current Measurement3/1 -> IBUSP/1
  Voltage Measurement3/1 -> VBUSP/1
  connections:
  Voltage Measurement3/LConn2 -- P-/RConn1
  L25/RConn1 -- (RLn)/2/RConn1
  (RL1.)/2/LConn1 -- L24/RConn1
  (RLn)/2/LConn1 -- Current Measurement3/RConn1 -- (RL1.)/2/RConn1
  Current Measurement3/LConn1 -- Voltage Measurement3/LConn1 -- P+/RConn1

== system MR30Simulinknodos/BUSP1 B21 ==
  (RL1.)/2 : powerlib/Elements/Series RLC Branch  LConnTagsString=__new0  RConnTagsString=__new0  BranchType=R  Resistance=0.165648/2  Inductance=1e-3  SetiL0=off  InitialCurrent=0  Capacitance=1e-6  Setx0=off  InitialVoltage=0  Measurements=None
  (RLn)/2 : powerlib/Elements/Series RLC Branch  LConnTagsString=__new0  RConnTagsString=__new0  BranchType=R  Resistance=0.496944/2  Inductance=1e-3  SetiL0=off  InitialCurrent=0  Capacitance=1e-6  Setx0=off  InitialVoltage=0  Measurements=None
  Current Measurement3 : powerlib/Measurements/Current Measurement  PhasorSimulation=off  OutputType=Complex  PSBequivalent=0
  Voltage Measurement3 : powerlib/Measurements/Voltage Measurement  PhasorSimulation=off  OutputType=Complex  PSBequivalent=0
  L29 : PMIOPort  Port=1  Side=Left
  P+ : PMIOPort  Port=2  Side=Right
  P- : PMIOPort  Port=3  Side=Right
  L27 : PMIOPort  Port=4  Side=Left
  IBUSP : Outport
  VBUSP : Outport  Port=2
  wires:
  Current Measurement3/1 -> IBUSP/1
  Voltage Measurement3/1 -> VBUSP/1
  connections:
  Voltage Measurement3/LConn2 -- P-/RConn1
  L27/RConn1 -- (RLn)/2/RConn1
  (RL1.)/2/LConn1 -- L29/RConn1
  (RLn)/2/LConn1 -- Current Measurement3/RConn1 -- (RL1.)/2/RConn1
  Current Measurement3/LConn1 -- Voltage Measurement3/LConn1 -- P+/RConn1

== system MR30Simulinknodos/BUSP1 B23 ==
  (RL1.)/2 : powerlib/Elements/Series RLC Branch  LConnTagsString=__new0  RConnTagsString=__new0  BranchType=R  Resistance=1.88496/2  Inductance=1e-3  SetiL0=off  InitialCurrent=0  Capacitance=1e-6  Setx0=off  InitialVoltage=0  Measurements=None
  (RLn)/2 : powerlib/Elements/Series RLC Branch  LConnTagsString=__new0  RConnTagsString=__new0  BranchType=R  Resistance=1.428/2  Inductance=1e-3  SetiL0=off  InitialCurrent=0  Capacitance=1e-6  Setx0=off  InitialVoltage=0  Measurements=None
  Current Measurement3 : powerlib/Measurements/Current Measurement  PhasorSimulation=off  OutputType=Complex  PSBequivalent=0
  Voltage Measurement3 : powerlib/Measurements/Voltage Measurement  PhasorSimulation=off  OutputType=Complex  PSBequivalent=0
  L32 : PMIOPort  Port=1  Side=Left
  P+ : PMIOPort  Port=2  Side=Right
  P- : PMIOPort  Port=3  Side=Right
  L30 : PMIOPort  Port=4  Side=Left
  IBUSP : Outport
  VBUSP : Outport  Port=2
  wires:
  Current Measurement3/1 -> IBUSP/1
  Voltage Measurement3/1 -> VBUSP/1
  connections:
  Voltage Measurement3/LConn2 -- P-/RConn1
  L30/RConn1 -- (RLn)/2/RConn1
  (RL1.)/2/LConn1 -- L32/RConn1
  (RLn)/2/LConn1 -- Current Measurement3/RConn1 -- (RL1.)/2/RConn1
  Current Measurement3/LConn1 -- Voltage Measurement3/LConn1 -- P+/RConn1

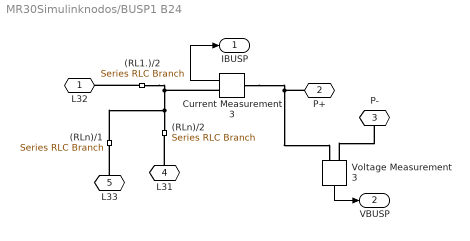
== system MR30Simulinknodos/BUSP1 B24 ==
  (RL1.)/2 : powerlib/Elements/Series RLC Branch  LConnTagsString=__new0  RConnTagsString=__new0  BranchType=R  Resistance=1.88496/2  Inductance=1e-3  SetiL0=off  InitialCurrent=0  Capacitance=1e-6  Setx0=off  InitialVoltage=0  Measurements=None
  (RLn)/1 : powerlib/Elements/Series RLC Branch  LConnTagsString=__new0  RConnTagsString=__new0  BranchType=R  Resistance=2.69178/2  Inductance=1e-3  SetiL0=off  InitialCurrent=0  Capacitance=1e-6  Setx0=off  InitialVoltage=0  Measurements=None
  (RLn)/2 : powerlib/Elements/Series RLC Branch  LConnTagsString=__new0  RConnTagsString=__new0  BranchType=R  Resistance=1.6422/2  Inductance=1e-3  SetiL0=off  InitialCurrent=0  Capacitance=1e-6  Setx0=off  InitialVoltage=0  Measurements=None
  Current Measurement3 : powerlib/Measurements/Current Measurement  PhasorSimulation=off  OutputType=Complex  PSBequivalent=0
  Voltage Measurement3 : powerlib/Measurements/Voltage Measurement  PhasorSimulation=off  OutputType=Complex  PSBequivalent=0
  L32 : PMIOPort  Port=1  Side=Left
  P+ : PMIOPort  Port=2  Side=Right
  P- : PMIOPort  Port=3  Side=Right
  L31 : PMIOPort  Port=4  Side=Left
  L33 : PMIOPort  Port=5  Side=Left
  IBUSP : Outport
  VBUSP : Outport  Port=2
  wires:
  Voltage Measurement3/1 -> VBUSP/1
  Current Measurement3/1 -> IBUSP/1
  connections:
  P+/RConn1 -- Voltage Measurement3/LConn1 -- Current Measurement3/LConn1
  (RL1.)/2/RConn1 -- Current Measurement3/RConn1 -- (RLn)/1/LConn1 -- (RLn)/2/LConn1
  (RL1.)/2/LConn1 -- L32/RConn1
  L31/RConn1 -- (RLn)/2/RConn1
  Voltage Measurement3/LConn2 -- P-/RConn1
  L33/RConn1 -- (RLn)/1/RConn1

== system MR30Simulinknodos/BUSP1 B26 ==
  (RLn)/2 : powerlib/Elements/Series RLC Branch  LConnTagsString=__new0  RConnTagsString=__new0  BranchType=R  Resistance=3.632832/2  Inductance=1e-3  SetiL0=off  InitialCurrent=0  Capacitance=1e-6  Setx0=off  InitialVoltage=0  Measurements=None
  Current Measurement3 : powerlib/Measurements/Current Measurement  PhasorSimulation=off  OutputType=Complex  PSBequivalent=0
  Voltage Measurement3 : powerlib/Measurements/Voltage Measurement  PhasorSimulation=off  OutputType=Complex  PSBequivalent=0
  P+ : PMIOPort  Port=1  Side=Right
  P- : PMIOPort  Port=2  Side=Right
  L34 : PMIOPort  Port=3  Side=Left
  IBUSP : Outport
  VBUSP : Outport  Port=2
  wires:
  Voltage Measurement3/1 -> VBUSP/1
  Current Measurement3/1 -> IBUSP/1
  connections:
  P+/RConn1 -- Voltage Measurement3/LConn1 -- Current Measurement3/LConn1
  Current Measurement3/RConn1 -- (RLn)/2/LConn1
  L34/RConn1 -- (RLn)/2/RConn1
  Voltage Measurement3/LConn2 -- P-/RConn1

== system MR30Simulinknodos/BUSP1 B29 ==
  (RL1.)/2 : powerlib/Elements/Series RLC Branch  LConnTagsString=__new0  RConnTagsString=__new0  BranchType=R  Resistance=3.138744/2  Inductance=1e-3  SetiL0=off  InitialCurrent=0  Capacitance=1e-6  Setx0=off  InitialVoltage=0  Measurements=None
  (RLn)/2 : powerlib/Elements/Series RLC Branch  LConnTagsString=__new0  RConnTagsString=__new0  BranchType=R  Resistance=3.425772/2  Inductance=1e-3  SetiL0=off  InitialCurrent=0  Capacitance=1e-6  Setx0=off  InitialVoltage=0  Measurements=None
  Current Measurement3 : powerlib/Measurements/Current Measurement  PhasorSimulation=off  OutputType=Complex  PSBequivalent=0
  Voltage Measurement3 : powerlib/Measurements/Voltage Measurement  PhasorSimulation=off  OutputType=Complex  PSBequivalent=0
  L37 : PMIOPort  Port=1  Side=Left
  P+ : PMIOPort  Port=2  Side=Right
  P- : PMIOPort  Port=3  Side=Right
  L39 : PMIOPort  Port=4  Side=Left
  IBUSP : Outport
  VBUSP : Outport  Port=2
  wires:
  Current Measurement3/1 -> IBUSP/1
  Voltage Measurement3/1 -> VBUSP/1
  connections:
  Voltage Measurement3/LConn2 -- P-/RConn1
  L39/RConn1 -- (RLn)/2/RConn1
  (RL1.)/2/LConn1 -- L37/RConn1
  (RLn)/2/LConn1 -- Current Measurement3/RConn1 -- (RL1.)/2/RConn1
  Current Measurement3/LConn1 -- Voltage Measurement3/LConn1 -- P+/RConn1

== system MR30Simulinknodos/BUSP1 B30 ==
  (RL1.)/2 : powerlib/Elements/Series RLC Branch  LConnTagsString=__new0  RConnTagsString=__new0  BranchType=R  Resistance=3.425772/2  Inductance=1e-3  SetiL0=off  InitialCurrent=0  Capacitance=1e-6  Setx0=off  InitialVoltage=0  Measurements=None
  (RLn)/2 : powerlib/Elements/Series RLC Branch  LConnTagsString=__new0  RConnTagsString=__new0  BranchType=R  Resistance=4.572456/2  Inductance=1e-3  SetiL0=off  InitialCurrent=0  Capacitance=1e-6  Setx0=off  InitialVoltage=0  Measurements=None
  Current Measurement3 : powerlib/Measurements/Current Measurement  PhasorSimulation=off  OutputType=Complex  PSBequivalent=0
  Voltage Measurement3 : powerlib/Measurements/Voltage Measurement  PhasorSimulation=off  OutputType=Complex  PSBequivalent=0
  L39 : PMIOPort  Port=1  Side=Left
  P+ : PMIOPort  Port=2  Side=Right
  P- : PMIOPort  Port=3  Side=Right
  L38 : PMIOPort  Port=4  Side=Left
  IBUSP : Outport
  VBUSP : Outport  Port=2
  wires:
  Voltage Measurement3/1 -> VBUSP/1
  Current Measurement3/1 -> IBUSP/1
  connections:
  P+/RConn1 -- Voltage Measurement3/LConn1 -- Current Measurement3/LConn1
  (RL1.)/2/RConn1 -- Current Measurement3/RConn1 -- (RLn)/2/LConn1
  (RL1.)/2/LConn1 -- L39/RConn1
  L38/RConn1 -- (RLn)/2/RConn1
  Voltage Measurement3/LConn2 -- P-/RConn1

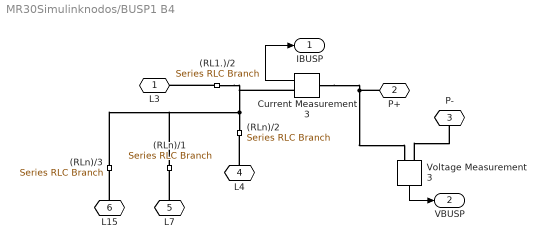
== system MR30Simulinknodos/BUSP1 B4 ==
  (RL1.)/2 : powerlib/Elements/Series RLC Branch  LConnTagsString=__new0  RConnTagsString=__new0  BranchType=R  Resistance=.81396/2  Inductance=1e-3  SetiL0=off  InitialCurrent=0  Capacitance=1e-6  Setx0=off  InitialVoltage=0  Measurements=None
  (RLn)/1 : powerlib/Elements/Series RLC Branch  LConnTagsString=__new0  RConnTagsString=__new0  BranchType=R  Resistance=0.169932/2  Inductance=1e-3  SetiL0=off  InitialCurrent=0  Capacitance=1e-6  Setx0=off  InitialVoltage=0  Measurements=None
  (RLn)/2 : powerlib/Elements/Series RLC Branch  LConnTagsString=__new0  RConnTagsString=__new0  BranchType=R  Resistance=.188496/2  Inductance=1e-3  SetiL0=off  InitialCurrent=0  Capacitance=1e-6  Setx0=off  InitialVoltage=0  Measurements=None
  (RLn)/3 : powerlib/Elements/Series RLC Branch  LConnTagsString=__new0  RConnTagsString=__new0  BranchType=R  Resistance=3.65568/2  Inductance=1e-3  SetiL0=off  InitialCurrent=0  Capacitance=1e-6  Setx0=off  InitialVoltage=0  Measurements=None
  Current Measurement3 : powerlib/Measurements/Current Measurement  PhasorSimulation=off  OutputType=Complex  PSBequivalent=0
  Voltage Measurement3 : powerlib/Measurements/Voltage Measurement  PhasorSimulation=off  OutputType=Complex  PSBequivalent=0
  L3 : PMIOPort  Port=1  Side=Left
  P+ : PMIOPort  Port=2  Side=Right
  P- : PMIOPort  Port=3  Side=Right
  L4 : PMIOPort  Port=4  Side=Left
  L7 : PMIOPort  Port=5  Side=Left
  L15 : PMIOPort  Port=6  Side=Right
  IBUSP : Outport
  VBUSP : Outport  Port=2
  wires:
  Current Measurement3/1 -> IBUSP/1
  Voltage Measurement3/1 -> VBUSP/1
  connections:
  Voltage Measurement3/LConn2 -- P-/RConn1
  L4/RConn1 -- (RLn)/2/RConn1
  (RL1.)/2/LConn1 -- L3/RConn1
  Current Measurement3/RConn1 -- (RL1.)/2/RConn1 -- (RLn)/3/LConn1 -- (RLn)/1/LConn1 -- (RLn)/2/LConn1
  Current Measurement3/LConn1 -- Voltage Measurement3/LConn1 -- P+/RConn1
  L7/RConn1 -- (RLn)/1/RConn1
  L15/RConn1 -- (RLn)/3/RConn1

== system MR30Simulinknodos/BUSP1 B7 ==
  (RL1.)/2 : powerlib/Elements/Series RLC Branch  LConnTagsString=__new0  RConnTagsString=__new0  BranchType=R  Resistance=.65688/2  Inductance=1e-3  SetiL0=off  InitialCurrent=0  Capacitance=1e-6  Setx0=off  InitialVoltage=0  Measurements=None
  (RLn)/2 : powerlib/Elements/Series RLC Branch  LConnTagsString=__new0  RConnTagsString=__new0  BranchType=R  Resistance=.381276/2  Inductance=1e-3  SetiL0=off  InitialCurrent=0  Capacitance=1e-6  Setx0=off  InitialVoltage=0  Measurements=None
  Current Measurement3 : powerlib/Measurements/Current Measurement  PhasorSimulation=off  OutputType=Complex  PSBequivalent=0
  Voltage Measurement3 : powerlib/Measurements/Voltage Measurement  PhasorSimulation=off  OutputType=Complex  PSBequivalent=0
  L8 : PMIOPort  Port=1  Side=Left
  P+ : PMIOPort  Port=2  Side=Right
  P- : PMIOPort  Port=3  Side=Right
  L9 : PMIOPort  Port=4  Side=Left
  IBUSP : Outport
  VBUSP : Outport  Port=2
  wires:
  Voltage Measurement3/1 -> VBUSP/1
  Current Measurement3/1 -> IBUSP/1
  connections:
  P+/RConn1 -- Voltage Measurement3/LConn1 -- Current Measurement3/LConn1
  (RL1.)/2/RConn1 -- Current Measurement3/RConn1 -- (RLn)/2/LConn1
  (RL1.)/2/LConn1 -- L8/RConn1
  L9/RConn1 -- (RLn)/2/RConn1
  Voltage Measurement3/LConn2 -- P-/RConn1

== system MR30Simulinknodos/BUSdroop B1 ==
  " (RL1)/2" : powerlib/Elements/Series RLC Branch  LConnTagsString=__new0  RConnTagsString=__new0  BranchType=R  Resistance=0.645456/2  Inductance=1e-3  SetiL0=off  InitialCurrent=0  Capacitance=1e-6  Setx0=off  InitialVoltage=0  Measurements=None
  " (RLn)/2" : powerlib/Elements/Series RLC Branch  LConnTagsString=__new0  RConnTagsString=__new0  BranchType=R  Resistance=0.274176/2  Inductance=1e-3  SetiL0=off  InitialCurrent=0  Capacitance=1e-6  Setx0=off  InitialVoltage=0  Measurements=None
  Current Measurement : powerlib/Measurements/Current Measurement  PhasorSimulation=off  OutputType=Complex  PSBequivalent=0
  Voltage Measurement : powerlib/Measurements/Voltage Measurement  PhasorSimulation=off  OutputType=Complex  PSBequivalent=0
  L2 : PMIOPort  Port=1  Side=Right
  DG1+ : PMIOPort  Port=2  Side=Left
  DG1- : PMIOPort  Port=3  Side=Left
  L1 : PMIOPort  Port=4  Side=Left
  VBUSdroop : Outport
  IBUSdroop : Outport  Port=2
  wires:
  Voltage Measurement/1 -> VBUSdroop/1
  Current Measurement/1 -> IBUSdroop/1
  connections:
  " (RL1)/2"/RConn1 -- L2/RConn1
  Current Measurement/LConn1 -- DG1+/RConn1 -- Voltage Measurement/LConn1
  " (RLn)/2"/LConn1 -- Current Measurement/RConn1 -- " (RL1)/2"/LConn1
  L1/RConn1 -- " (RLn)/2"/RConn1
  Voltage Measurement/LConn2 -- DG1-/RConn1

== system MR30Simulinknodos/BUSdroop B11 ==
  " (RL1)/2" : powerlib/Elements/Series RLC Branch  LConnTagsString=__new0  RConnTagsString=__new0  BranchType=R  Resistance=2.97024/2  Inductance=1e-3  SetiL0=off  InitialCurrent=0  Capacitance=1e-6  Setx0=off  InitialVoltage=0  Measurements=None
  Current Measurement : powerlib/Measurements/Current Measurement  PhasorSimulation=off  OutputType=Complex  PSBequivalent=0
  Voltage Measurement : powerlib/Measurements/Voltage Measurement  PhasorSimulation=off  OutputType=Complex  PSBequivalent=0
  L13 : PMIOPort  Port=1  Side=Right
  DG5+ : PMIOPort  Port=2  Side=Left
  DG5- : PMIOPort  Port=3  Side=Left
  VBUSdroop : Outport
  IBUSdroop : Outport  Port=2
  wires:
  Current Measurement/1 -> IBUSdroop/1
  Voltage Measurement/1 -> VBUSdroop/1
  connections:
  Voltage Measurement/LConn2 -- DG5-/RConn1
  " (RL1)/2"/LConn1 -- Current Measurement/RConn1
  Voltage Measurement/LConn1 -- DG5+/RConn1 -- Current Measurement/LConn1
  " (RL1)/2"/RConn1 -- L13/RConn1

== system MR30Simulinknodos/BUSdroop B13 ==
  " (RLn)/2" : powerlib/Elements/Series RLC Branch  LConnTagsString=__new0  RConnTagsString=__new0  BranchType=R  Resistance=1.9992/2  Inductance=1e-3  SetiL0=off  InitialCurrent=0  Capacitance=1e-6  Setx0=off  InitialVoltage=0  Measurements=None
  Current Measurement : powerlib/Measurements/Current Measurement  PhasorSimulation=off  OutputType=Complex  PSBequivalent=0
  Voltage Measurement : powerlib/Measurements/Voltage Measurement  PhasorSimulation=off  OutputType=Complex  PSBequivalent=0
  DG1+ : PMIOPort  Port=1  Side=Left
  DG1- : PMIOPort  Port=2  Side=Left
  L16 : PMIOPort  Port=3  Side=Left
  VBUSdroop : Outport
  IBUSdroop : Outport  Port=2
  wires:
  Voltage Measurement/1 -> VBUSdroop/1
  Current Measurement/1 -> IBUSdroop/1
  connections:
  Current Measurement/LConn1 -- DG1+/RConn1 -- Voltage Measurement/LConn1
  " (RLn)/2"/LConn1 -- Current Measurement/RConn1
  L16/RConn1 -- " (RLn)/2"/RConn1
  Voltage Measurement/LConn2 -- DG1-/RConn1

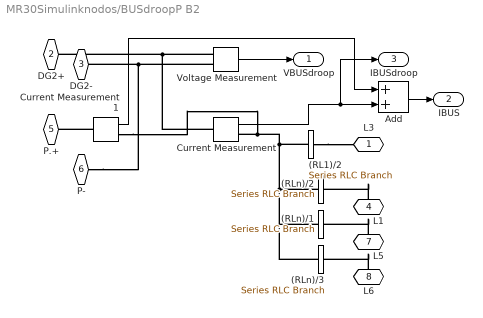
== system MR30Simulinknodos/BUSdroopP B2 ==
  " (RL1)/2" : powerlib/Elements/Series RLC Branch  LConnTagsString=__new0  RConnTagsString=__new0  BranchType=R  Resistance=.81396/2  Inductance=1e-3  SetiL0=off  InitialCurrent=0  Capacitance=1e-6  Setx0=off  InitialVoltage=0  Measurements=None
  " (RLn)/1" : powerlib/Elements/Series RLC Branch  LConnTagsString=__new0  RConnTagsString=__new0  BranchType=R  Resistance=.674016/2  Inductance=1e-3  SetiL0=off  InitialCurrent=0  Capacitance=1e-6  Setx0=off  InitialVoltage=0  Measurements=None
  " (RLn)/2" : powerlib/Elements/Series RLC Branch  LConnTagsString=__new0  RConnTagsString=__new0  BranchType=R  Resistance=0.274176/2  Inductance=1e-3  SetiL0=off  InitialCurrent=0  Capacitance=1e-6  Setx0=off  InitialVoltage=0  Measurements=None
  " (RLn)/3" : powerlib/Elements/Series RLC Branch  LConnTagsString=__new0  RConnTagsString=__new0  BranchType=R  Resistance=.829668/2  Inductance=1e-3  SetiL0=off  InitialCurrent=0  Capacitance=1e-6  Setx0=off  InitialVoltage=0  Measurements=None
  Add : Sum
  Current Measurement : powerlib/Measurements/Current Measurement  PhasorSimulation=off  OutputType=Complex  PSBequivalent=0
  Current Measurement1 : powerlib/Measurements/Current Measurement  PhasorSimulation=off  OutputType=Complex  PSBequivalent=0
  Voltage Measurement : powerlib/Measurements/Voltage Measurement  PhasorSimulation=off  OutputType=Complex  PSBequivalent=0
  L3 : PMIOPort  Port=1  Side=Right
  DG2+ : PMIOPort  Port=2  Side=Left
  DG2- : PMIOPort  Port=3  Side=Left
  L1 : PMIOPort  Port=4  Side=Left
  P.+ : PMIOPort  Port=5  Side=Right
  P- : PMIOPort  Port=6  Side=Right
  L5 : PMIOPort  Port=7  Side=Left
  L6 : PMIOPort  Port=8  Side=Right
  VBUSdroop : Outport
  IBUS : Outport  Port=2
  IBUSdroop : Outport  Port=3
  wires:
  Voltage Measurement/1 -> VBUSdroop/1
  Current Measurement1/1 -> Add/1
  Add/1 -> IBUS/1
  Current Measurement/1 -> IBUSdroop/1, Add/2
  connections:
  Voltage Measurement/LConn2 -- P-/RConn1 -- DG2-/RConn1
  L1/RConn1 -- " (RLn)/2"/RConn1
  " (RL1)/2"/LConn1 -- " (RLn)/3"/LConn1 -- " (RLn)/1"/LConn1 -- " (RLn)/2"/LConn1 -- Current Measurement1/RConn1 -- Current Measurement/RConn1
  Voltage Measurement/LConn1 -- DG2+/RConn1 -- Current Measurement/LConn1
  " (RL1)/2"/RConn1 -- L3/RConn1
  L5/RConn1 -- " (RLn)/1"/RConn1
  L6/RConn1 -- " (RLn)/3"/RConn1
  Current Measurement1/LConn1 -- P.+/RConn1

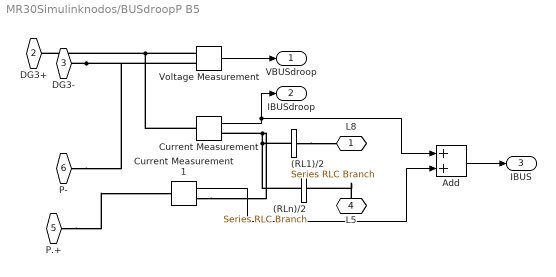
== system MR30Simulinknodos/BUSdroopP B5 ==
  " (RL1)/2" : powerlib/Elements/Series RLC Branch  LConnTagsString=__new0  RConnTagsString=__new0  BranchType=R  Resistance=.65688/2  Inductance=1e-3  SetiL0=off  InitialCurrent=0  Capacitance=1e-6  Setx0=off  InitialVoltage=0  Measurements=None
  " (RLn)/2" : powerlib/Elements/Series RLC Branch  LConnTagsString=__new0  RConnTagsString=__new0  BranchType=R  Resistance=.674016/2  Inductance=1e-3  SetiL0=off  InitialCurrent=0  Capacitance=1e-6  Setx0=off  InitialVoltage=0  Measurements=None
  Add : Sum
  Current Measurement : powerlib/Measurements/Current Measurement  PhasorSimulation=off  OutputType=Complex  PSBequivalent=0
  Current Measurement1 : powerlib/Measurements/Current Measurement  PhasorSimulation=off  OutputType=Complex  PSBequivalent=0
  Voltage Measurement : powerlib/Measurements/Voltage Measurement  PhasorSimulation=off  OutputType=Complex  PSBequivalent=0
  L8 : PMIOPort  Port=1  Side=Right
  DG3+ : PMIOPort  Port=2  Side=Left
  DG3- : PMIOPort  Port=3  Side=Left
  L5 : PMIOPort  Port=4  Side=Left
  P.+ : PMIOPort  Port=5  Side=Right
  P- : PMIOPort  Port=6  Side=Right
  VBUSdroop : Outport
  IBUSdroop : Outport  Port=2
  IBUS : Outport  Port=3
  wires:
  Voltage Measurement/1 -> VBUSdroop/1
  Current Measurement/1 -> Add/1, IBUSdroop/1
  Current Measurement1/1 -> Add/2
  Add/1 -> IBUS/1
  connections:
  " (RL1)/2"/RConn1 -- L8/RConn1
  Current Measurement/LConn1 -- DG3+/RConn1 -- Voltage Measurement/LConn1
  " (RLn)/2"/LConn1 -- Current Measurement/RConn1 -- Current Measurement1/RConn1 -- " (RL1)/2"/LConn1
  L5/RConn1 -- " (RLn)/2"/RConn1
  DG3-/RConn1 -- P-/RConn1 -- Voltage Measurement/LConn2
  P.+/RConn1 -- Current Measurement1/LConn1

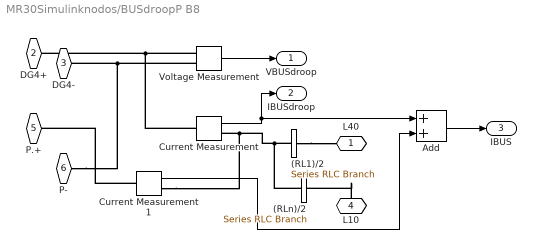
== system MR30Simulinknodos/BUSdroopP B8 ==
  " (RL1)/2" : powerlib/Elements/Series RLC Branch  LConnTagsString=__new0  RConnTagsString=__new0  BranchType=R  Resistance=0.908208/2  Inductance=1e-3  SetiL0=off  InitialCurrent=0  Capacitance=1e-6  Setx0=off  InitialVoltage=0  Measurements=None
  " (RLn)/2" : powerlib/Elements/Series RLC Branch  LConnTagsString=__new0  RConnTagsString=__new0  BranchType=R  Resistance=.17136/2  Inductance=1e-3  SetiL0=off  InitialCurrent=0  Capacitance=1e-6  Setx0=off  InitialVoltage=0  Measurements=None
  Add : Sum
  Current Measurement : powerlib/Measurements/Current Measurement  PhasorSimulation=off  OutputType=Complex  PSBequivalent=0
  Current Measurement1 : powerlib/Measurements/Current Measurement  PhasorSimulation=off  OutputType=Complex  PSBequivalent=0
  Voltage Measurement : powerlib/Measurements/Voltage Measurement  PhasorSimulation=off  OutputType=Complex  PSBequivalent=0
  L40 : PMIOPort  Port=1  Side=Right
  DG4+ : PMIOPort  Port=2  Side=Left
  DG4- : PMIOPort  Port=3  Side=Left
  L10 : PMIOPort  Port=4  Side=Left
  P.+ : PMIOPort  Port=5  Side=Right
  P- : PMIOPort  Port=6  Side=Right
  VBUSdroop : Outport
  IBUSdroop : Outport  Port=2
  IBUS : Outport  Port=3
  wires:
  Voltage Measurement/1 -> VBUSdroop/1
  Current Measurement/1 -> Add/1, IBUSdroop/1
  Current Measurement1/1 -> Add/2
  Add/1 -> IBUS/1
  connections:
  Voltage Measurement/LConn2 -- P-/RConn1 -- DG4-/RConn1
  L10/RConn1 -- " (RLn)/2"/RConn1
  " (RL1)/2"/LConn1 -- Current Measurement1/RConn1 -- Current Measurement/RConn1 -- " (RLn)/2"/LConn1
  Voltage Measurement/LConn1 -- DG4+/RConn1 -- Current Measurement/LConn1
  " (RL1)/2"/RConn1 -- L40/RConn1
  Current Measurement1/LConn1 -- P.+/RConn1

== system MR30Simulinknodos/BUSstep B22 ==
  " (RL1)/2" : powerlib/Elements/Series RLC Branch  LConnTagsString=__new0  RConnTagsString=__new0  BranchType=R  Resistance=1.6422/2  Inductance=1e-3  SetiL0=off  InitialCurrent=0  Capacitance=1e-6  Setx0=off  InitialVoltage=0  Measurements=None
  " (RL2)/2" : powerlib/Elements/Series RLC Branch  LConnTagsString=__new0  RConnTagsString=__new0  BranchType=R  Resistance=0.165648/2  Inductance=1e-3  SetiL0=off  InitialCurrent=0  Capacitance=1e-6  Setx0=off  InitialVoltage=0  Measurements=None
  " (RLn)/2" : powerlib/Elements/Series RLC Branch  LConnTagsString=__new0  RConnTagsString=__new0  BranchType=R  Resistance=1.038156/2  Inductance=1e-3  SetiL0=off  InitialCurrent=0  Capacitance=1e-6  Setx0=off  InitialVoltage=0  Measurements=None
  Ground : powerlib/Elements/Ground  LConnTagsString=a
  Voltage Measurement : powerlib/Measurements/Voltage Measurement  PhasorSimulation=off  OutputType=Complex  PSBequivalent=0
  L31 : PMIOPort  Port=1  Side=Right
  L29 : PMIOPort  Port=2  Side=Left
  L28 : PMIOPort  Port=3  Side=Left
  VBUSstep : Outport
  wires:
  Voltage Measurement/1 -> VBUSstep/1
  connections:
  " (RL1)/2"/RConn1 -- L31/RConn1
  " (RL2)/2"/LConn1 -- L29/RConn1
  Ground/LConn1 -- Voltage Measurement/LConn2
  Voltage Measurement/LConn1 -- " (RLn)/2"/LConn1 -- " (RL2)/2"/RConn1 -- " (RL1)/2"/LConn1
  L28/RConn1 -- " (RLn)/2"/RConn1
